simulink model "EV_model"  (R2020a)
settings: Solver=VariableStepAuto  StartTime=0  StopTime=length_DriveCycle* n_repeat  FixedStep=1  RelTol=1e-3
model workspace (MAT data in the model file):
  Af = 4
  Cd = 0.3
  DrCycles : object (value not decoded)
  I = 1
  Kbr = 5000
  P = 20
  TimeHWFET = 765
  TimeUDDS = 1372
  TimeUS06 = 596
  axle_b = 10
  axle_k = 5000
  bevAxle_wc = 400
  bevNp = 2
  bevNs = 30
  diffRatio = 3.4
  diffRatio1 = 3.4
  motorMaxTorqueNm = [500 500 500 500 500 500 416.666666667 357.142857143 312.5 277.777777778 250 227.272727273 ... (16 elements, 1x16)]
  motorSpeedRadPs = [0 40 80 120 160 200 240 280 320 360 400 440 ... (16 elements, 1x16)]
  vehicleMass = 1500
  wheelRadius = 0.35
values from neighbouring files (symbols this model uses):
  b = 4.48/2    (= 2.24)    [NissanLeaf_input_data.m]    (also in TeslaS_input_data.m = 2.5)
  Ct = Cp_cell*rho_cell*cell_volume    (= 2759947.2)    [NissanLeaf_input_data.m]    (also in TeslaS_input_data.m = 37.7660192772)
  driving_range = 363    [NissanLeaf_input_data.m]    (also in TeslaS_input_data.m = 600)
  m = 1789    [NissanLeaf_input_data.m]    (also in TeslaS_input_data.m = 2250)
  motorMaxTorqueNm_my = [340 340 340 340 340 340 300 260  230  210 190   175 160 150 140 130 125 120]    [NissanLeaf_input_data.m]    (also in TeslaS_input_data.m = [660 660 660 660 660 660 550 475 400 325 275 225 200 175 150)
  motorSpeedRadPs_my = [1000 1500 2000 2500 3000 3250 3500 4000 4500 5000 5500 6000 6500  7000 7500 8000 8500 9000]*transRatio*2*pi/60    [NissanLeaf_input_data.m]    (also in TeslaS_input_data.m = [0 10 20 30 40 50 60 70 80 90 100 110 120 130 140 150]*0.447)
  regen_eff = 0.7    [NissanLeaf_input_data.m]    (also in TeslaS_input_data.m)
  Rt = 0.01    [NissanLeaf_input_data.m]    (also in TeslaS_input_data.m = 0.316348525327)
  T = 20    [NissanLeaf_input_data.m]    (also in TeslaS_input_data.m = 25; battery_parametrization.m)
  transRatio = 8.19    [NissanLeaf_input_data.m]    (also in TeslaS_input_data.m = 9.3)
undefined symbols (not defined in the file or in its folder): Driver, Wheels_Driver_VehDyn_Lib
libraries: autolibshared x3, simulink x2, autolibdatasheetbattery x1, autolibmappedmotor x1, autolibsharedcoupling x1, autolibshareddiff x1
(part 3 of 3)

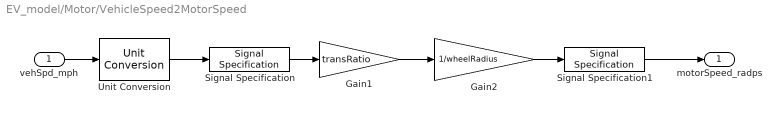
== system EV_model/Motor/VehicleSpeed2MotorSpeed ==
  vehSpd_mph : Inport
  Gain1 : Gain  Gain=transRatio
  Gain2 : Gain  Gain=1/wheelRadius
  Signal Specification : SignalSpecification  Unit=m/s
  Signal Specification1 : SignalSpecification  Unit=rad/s
  Unit Conversion : UnitConversion
  motorSpeed_radps : Outport  VectorParamsAs1DForOutWhenUnconnected=off
  wires:
  Signal Specification1/1 -> motorSpeed_radps/1
  Unit Conversion/1 -> Signal Specification/1
  vehSpd_mph/1 -> Unit Conversion/1
  Signal Specification/1 -> Gain1/1
  Gain1/1 -> Gain2/1
  Gain2/1 -> Signal Specification1/1

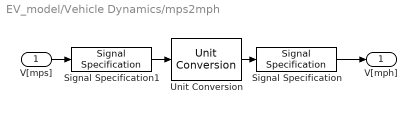
== system EV_model/Vehicle Dynamics/mps2mph ==
  V[mps] : Inport
  Signal Specification : SignalSpecification  Unit=mph
  Signal Specification1 : SignalSpecification  Unit=m/s
  Unit Conversion : UnitConversion
  V[mph] : Outport  VectorParamsAs1DForOutWhenUnconnected=off
  wires:
  Signal Specification/1 -> V[mph]/1
  Signal Specification1/1 -> Unit Conversion/1
  Unit Conversion/1 -> Signal Specification/1
  V[mps]/1 -> Signal Specification1/1
